simulink model "algebraicContaint"  (R2024b)
settings: Solver=VariableStepAuto  StartTime=0.0  StopTime=10.0  RelTol=1e-3
settings Model: Creator=optimus  LastModifiedBy=optimus

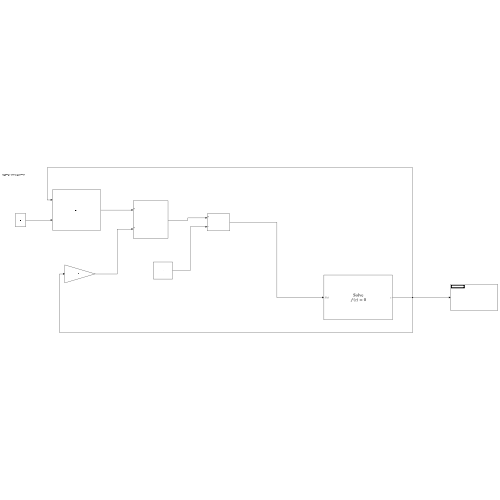
[thumbnail: Simulink's stored preview of the top-level diagram]
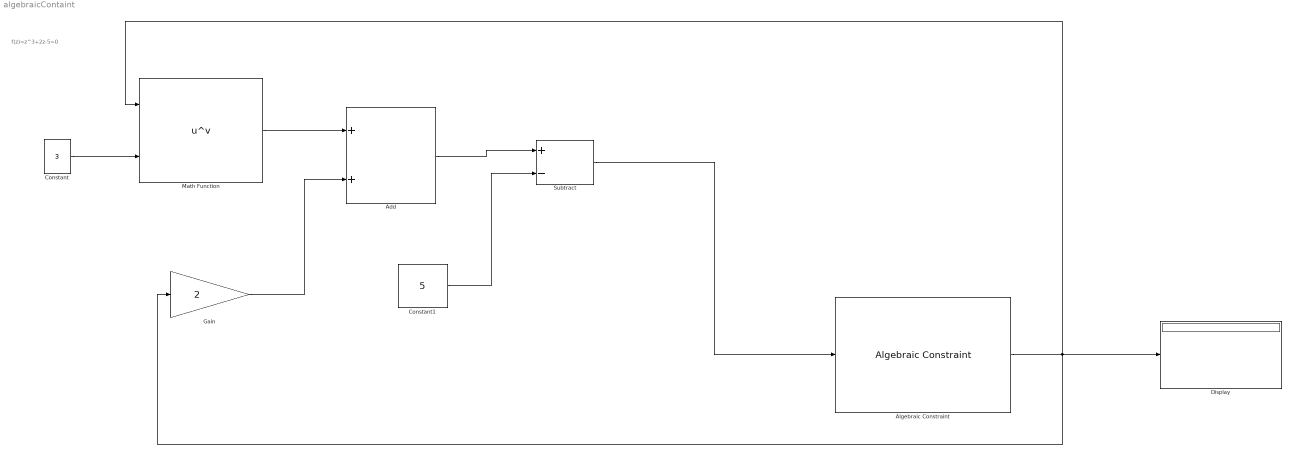
== system algebraicContaint ==
  note: f(z)=z^3+2z-5=0
  Add : Sum
  Algebraic Constraint : AlgebraicConstraint
  Constant : Constant  Value=3
  Constant1 : Constant  Value=5
  Display : Display
  Gain : Gain  Gain=2
  Math Function : Math  Operator=pow
  Subtract : Sum  Inputs=+-
  wires:
  Algebraic Constraint/1 -> Math Function/1, Gain/1, Display/1
  Math Function/1 -> Add/1
  Constant/1 -> Math Function/2
  Gain/1 -> Add/2
  Add/1 -> Subtract/1
  Subtract/1 -> Algebraic Constraint/1
  Constant1/1 -> Subtract/2
